simulink model "p_regulator"  (R2022b)
settings: Solver=ode45  StartTime=0.0  StopTime=25  MaxStep=0.03  RelTol=1e-4
values from neighbouring files (symbols this model uses):
  B = 0.120    (= 0.12)    [run_all.m]    (also in run_all_litle.m)
  K_r = 2    [run_all.m]    (also in run_all_litle.m)
  K_s = 0.5    [run_all.m]    (also in run_all_litle.m)
  MAX_U = 50.0    (= 50)    [run_all.m]    (also in run_all_litle.m)
  r = 0.029    [run_all.m]    (also in run_all_litle.m)
settings Model: Creator=Eternal_Core  LastModifiedBy=Eternal_Core

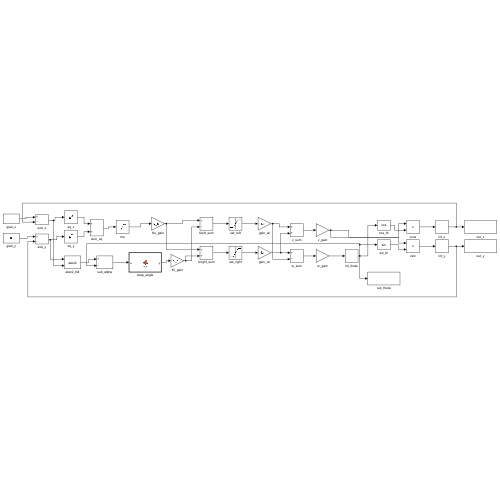
[thumbnail: Simulink's stored preview of the top-level diagram]
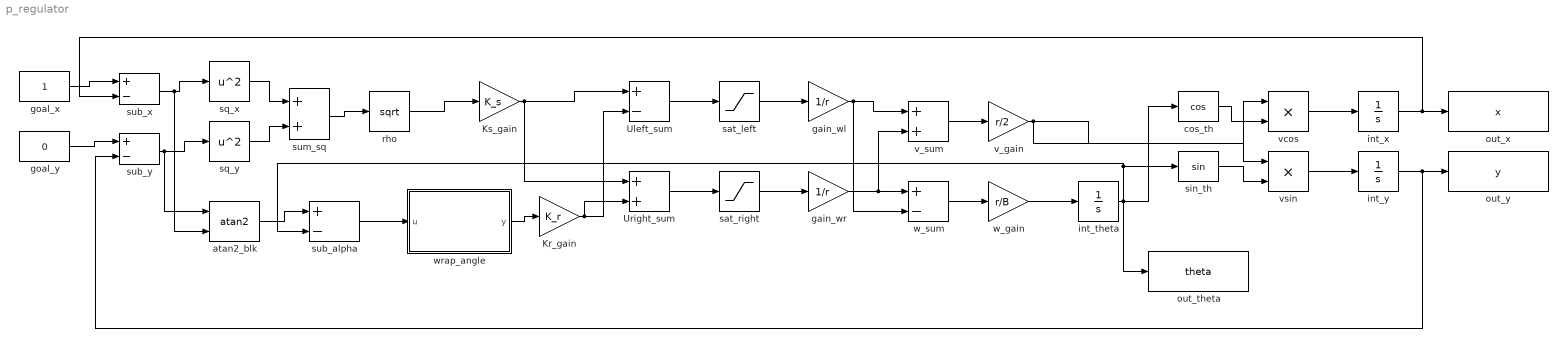
== system p_regulator ==
  Kr_gain : Gain  Gain=K_r
  Ks_gain : Gain  Gain=K_s
  Uleft_sum : Sum  Inputs=+-
  Uright_sum : Sum
  atan2_blk : Trigonometry  Operator=atan2
  cos_th : Trigonometry  Operator=cos
  gain_wl : Gain  Gain=1/r
  gain_wr : Gain  Gain=1/r
  goal_x : Constant
  goal_y : Constant  Value=0
  int_theta : Integrator
  int_x : Integrator
  int_y : Integrator
  out_theta : ToWorkspace  VariableName=theta  SaveFormat=Timeseries  SampleTime=-1
  out_x : ToWorkspace  VariableName=x  SaveFormat=Timeseries  SampleTime=-1
  out_y : ToWorkspace  VariableName=y  SaveFormat=Timeseries  SampleTime=-1
  rho : Sqrt
  sat_left : Saturate  UpperLimit=MAX_U  LowerLimit=-MAX_U
  sat_right : Saturate  UpperLimit=MAX_U  LowerLimit=-MAX_U
  sin_th : Trigonometry
  sq_x : Math  Operator=square
  sq_y : Math  Operator=square
  sub_alpha : Sum  Inputs=+-
  sub_x : Sum  Inputs=+-
  sub_y : Sum  Inputs=+-
  sum_sq : Sum
  v_gain : Gain  Gain=r/2
  v_sum : Sum
  vcos : Product
  vsin : Product
  w_gain : Gain  Gain=r/B
  w_sum : Sum  Inputs=+-
  wrap_angle : MATLAB Function  TreatAsAtomicUnit=on
  wires:
  goal_x/1 -> sub_x/1
  goal_y/1 -> sub_y/1
  sub_x/1 -> sq_x/1, atan2_blk/2
  sub_y/1 -> sq_y/1, atan2_blk/1
  sq_x/1 -> sum_sq/1
  sq_y/1 -> sum_sq/2
  sum_sq/1 -> rho/1
  atan2_blk/1 -> sub_alpha/1
  sub_alpha/1 -> wrap_angle/1(u)
  rho/1 -> Ks_gain/1
  wrap_angle/1(y) -> Kr_gain/1
  Ks_gain/1 -> Uleft_sum/1, Uright_sum/1
  Kr_gain/1 -> Uleft_sum/2, Uright_sum/2
  Uleft_sum/1 -> sat_left/1
  Uright_sum/1 -> sat_right/1
  sat_left/1 -> gain_wl/1
  sat_right/1 -> gain_wr/1
  gain_wl/1 -> v_sum/1, w_sum/2
  gain_wr/1 -> v_sum/2, w_sum/1
  v_sum/1 -> v_gain/1
  w_sum/1 -> w_gain/1
  w_gain/1 -> int_theta/1
  int_theta/1 -> sin_th/1, sub_alpha/2, cos_th/1, out_theta/1
  v_gain/1 -> vcos/1, vsin/1
  cos_th/1 -> vcos/2
  sin_th/1 -> vsin/2
  vcos/1 -> int_x/1
  vsin/1 -> int_y/1
  int_x/1 -> sub_x/2, out_x/1
  int_y/1 -> sub_y/2, out_y/1

== matlab function p_regulator/wrap_angle ==
  data: u input; y output
function y = fcn(u)
y = u;
while y > pi
  y = y - 2*pi;
end
while y < -pi
  y = y + 2*pi;
end
